simulink model "punto2c"  (R2018b)
settings: Solver=VariableStepAuto  StartTime=0  StopTime=8  RelTol=1e-3
libraries: dspsrcs4 x1
settings Model: Creator=carta  LastModifiedBy=michha

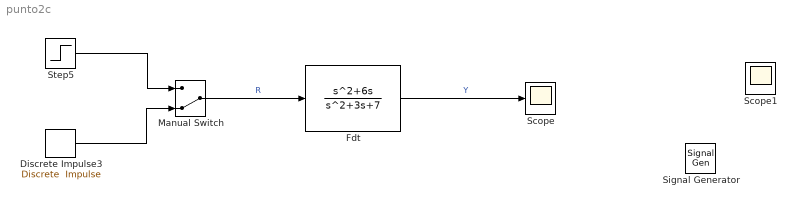
== system punto2c ==
  Discrete Impulse3 : dspsrcs4/Discrete  Impulse  Delay=0  SampleTime=0.1  FrameSample=1  OutputFrames=off  dataType=double  isSigned=on  wordLen=16  udDataType=sfix(16)  fracBitsMode=Best precision  numFracBits=15  OutDataTypeStr=double  LastOutDataTypeStr=double
  Fdt : TransferFcn  Numerator=[1 6 0]  Denominator=[1 3 7]
  Manual Switch : ManualSwitch  CurrentSetting=0
  Scope : Scope
  Step5 : Step  Time=0  SampleTime=0
  Scope1 : Scope
  Signal Generator : SignalGenerator  IOType=siggen
  wires:
  Fdt/1 -> Scope/1  "Y"
  Manual Switch/1 -> Fdt/1  "R"
  Discrete Impulse3/1 -> Manual Switch/2
  Step5/1 -> Manual Switch/1
